simulink model "orbitCtrl_params_test"  (R2023b)
settings: Solver=VariableStepAuto  StartTime=0.0  StopTime=5000  FixedStep=0.1  RelTol=1e-12  AbsTol=1e-13
undefined symbols (not defined in the file): v0, x0
libraries: dyn_lib x2
settings Model: Creator=brent  LastModifiedBy=brent

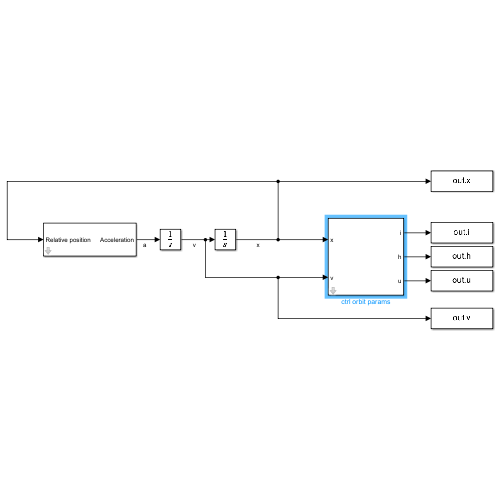
[thumbnail: Simulink's stored preview of the top-level diagram]
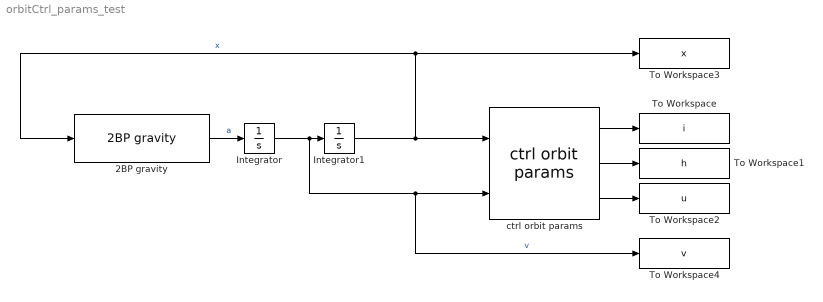
== system orbitCtrl_params_test ==
  2BP gravity : dyn_lib/2BP gravity  mu=398600
      settings: SourceProductName=Dynamics library
  Integrator : Integrator  InitialCondition=v0
  Integrator1 : Integrator  InitialCondition=x0
  To Workspace : ToWorkspace  VariableName=i  SampleTime=-1
      settings: Save2DSignal=2-D array (concatenate along first dimension)
  To Workspace1 : ToWorkspace  VariableName=h  SampleTime=-1
      settings: Save2DSignal=2-D array (concatenate along first dimension)
  To Workspace2 : ToWorkspace  VariableName=u  SampleTime=-1
      settings: Save2DSignal=2-D array (concatenate along first dimension)
  To Workspace3 : ToWorkspace  VariableName=x  SampleTime=-1
  To Workspace4 : ToWorkspace  VariableName=v  SampleTime=-1
  ctrl orbit params : dyn_lib/ctrl orbit params
      settings: SourceProductName=Dynamics library
  wires:
  2BP gravity/1 -> Integrator/1  "a"
  Integrator/1 -> To Workspace4/1, ctrl orbit params/2, Integrator1/1  "v"
  Integrator1/1 -> To Workspace3/1, 2BP gravity/1, ctrl orbit params/1  "x"
  ctrl orbit params/1 -> To Workspace/1
  ctrl orbit params/2 -> To Workspace1/1
  ctrl orbit params/3 -> To Workspace2/1
